simulink model "cluster_robot_control_7_rotation_sim"  (R2016a)
settings: Solver=ode5  StartTime=0.0  StopTime=100  FixedStep=0.001  RelTol=1e-3
values from neighbouring files (symbols this model uses):
  E = eye(8)    [cluster_robot_control_7_rotation.m]    (also in cluster_robot_control_8_final.m)
  LK1 = -LK1    [cluster_robot_control_7_rotation.m]    (also in cluster_robot_control_8_final.m)
  v0 = [1 1 2 1 1 1 1 1]'    [cluster_robot_control_7_rotation.m]    (also in cluster_robot_control_8_final.m)
  w0 = 1    [cluster_robot_control_7_rotation.m]    (also in cluster_robot_control_8_final.m)
  x0 = [1 3 2 1 3 2 4 5]'    [cluster_robot_control_7_rotation.m]    (also in cluster_robot_control_8_final.m)
  xd = [0 0 0 0 0 0 0 0]    [cluster_robot_control_7_rotation.m]    (also in cluster_robot_control_8_final.m)
settings Model: Creator=richa  LastModifiedBy=richa

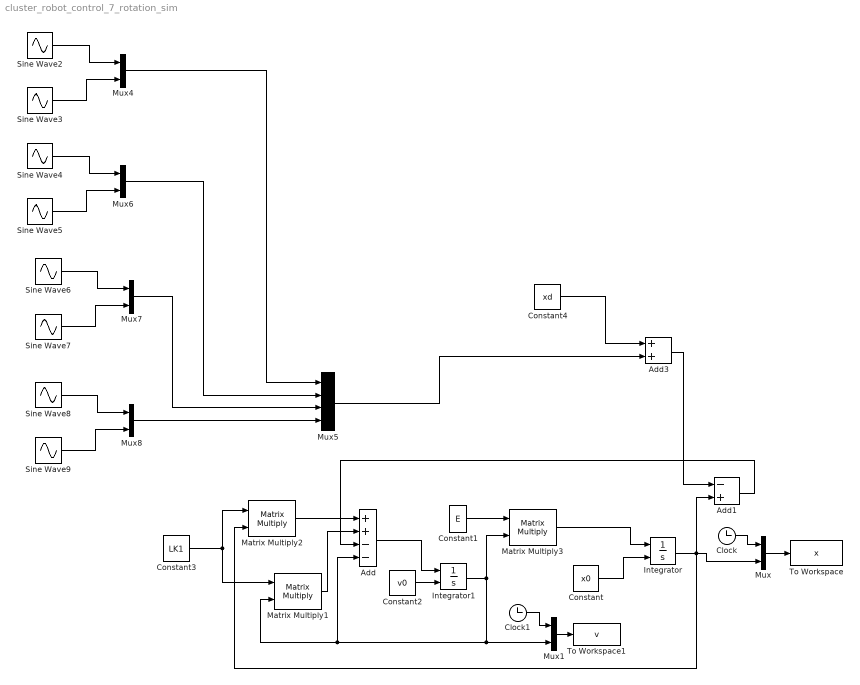
== system cluster_robot_control_7_rotation_sim ==
  Add : Sum  Inputs=++--
  Add1 : Sum  Inputs=-+
  Add3 : Sum
  Clock : Clock
  Clock1 : Clock
  Constant : Constant  Value=x0
  Constant1 : Constant  Value=E
  Constant2 : Constant  Value=v0
  Constant3 : Constant  Value=LK1
  Constant4 : Constant  Value=xd
  Integrator : Integrator  InitialConditionSource=external
  Integrator1 : Integrator  InitialConditionSource=external
  Matrix Multiply1 : Product  Multiplication=Matrix(*)
  Matrix Multiply2 : Product  Multiplication=Matrix(*)
  Matrix Multiply3 : Product  Multiplication=Matrix(*)
  Mux{,1,4,6..8} (6 alike) : Mux  Inputs=2
  Mux5 : Mux
  Sine Wave2 : Sin  Amplitude=100  Frequency=w0  SampleTime=0
  Sine Wave3 : Sin  Amplitude=100  Frequency=w0  Phase=pi/2  SampleTime=0
  Sine Wave4 : Sin  Amplitude=100  Frequency=w0  Phase=pi/2  SampleTime=0
  Sine Wave5 : Sin  Amplitude=100  Frequency=w0  Phase=pi  SampleTime=0
  Sine Wave6 : Sin  Amplitude=100  Frequency=w0  Phase=pi  SampleTime=0
  Sine Wave7 : Sin  Amplitude=100  Frequency=w0  Phase=pi*3/2  SampleTime=0
  Sine Wave8 : Sin  Amplitude=100  Frequency=w0  Phase=pi*3/2  SampleTime=0
  Sine Wave9 : Sin  Amplitude=100  Frequency=w0  Phase=2*pi  SampleTime=0
  To Workspace : ToWorkspace  VariableName=x  SampleTime=-1
  To Workspace1 : ToWorkspace  VariableName=v  SampleTime=-1
  wires:
  Constant/1 -> Integrator/2
  Mux/1 -> To Workspace/1
  Clock/1 -> Mux/1
  Constant2/1 -> Integrator1/2
  Constant3/1 -> Matrix Multiply1/1, Matrix Multiply2/1
  Mux1/1 -> To Workspace1/1
  Clock1/1 -> Mux1/1
  Matrix Multiply2/1 -> Add/1
  Matrix Multiply1/1 -> Add/2
  Add/1 -> Integrator1/1
  Constant1/1 -> Matrix Multiply3/1
  Matrix Multiply3/1 -> Integrator/1
  Add1/1 -> Add/3
  Integrator/1 -> Matrix Multiply2/2, Add1/2, Mux/2
  Integrator1/1 -> Matrix Multiply3/2, Matrix Multiply1/2, Add/4, Mux1/2
  Add3/1 -> Add1/1
  Sine Wave2/1 -> Mux4/1
  Sine Wave3/1 -> Mux4/2
  Mux4/1 -> Mux5/1
  Mux5/1 -> Add3/2
  Sine Wave4/1 -> Mux6/1
  Sine Wave5/1 -> Mux6/2
  Sine Wave6/1 -> Mux7/1
  Sine Wave7/1 -> Mux7/2
  Sine Wave8/1 -> Mux8/1
  Sine Wave9/1 -> Mux8/2
  Mux6/1 -> Mux5/2
  Mux7/1 -> Mux5/3
  Mux8/1 -> Mux5/4
  Constant4/1 -> Add3/1
